simulink model "washout6"  (R2018b)
settings: Solver=VariableStepAuto  StartTime=0.0  StopTime=50  RelTol=1e-3
libraries: simulink x1, fuzblock x1, cstblocks x1
settings Model: Creator=15705  LastModifiedBy=15705

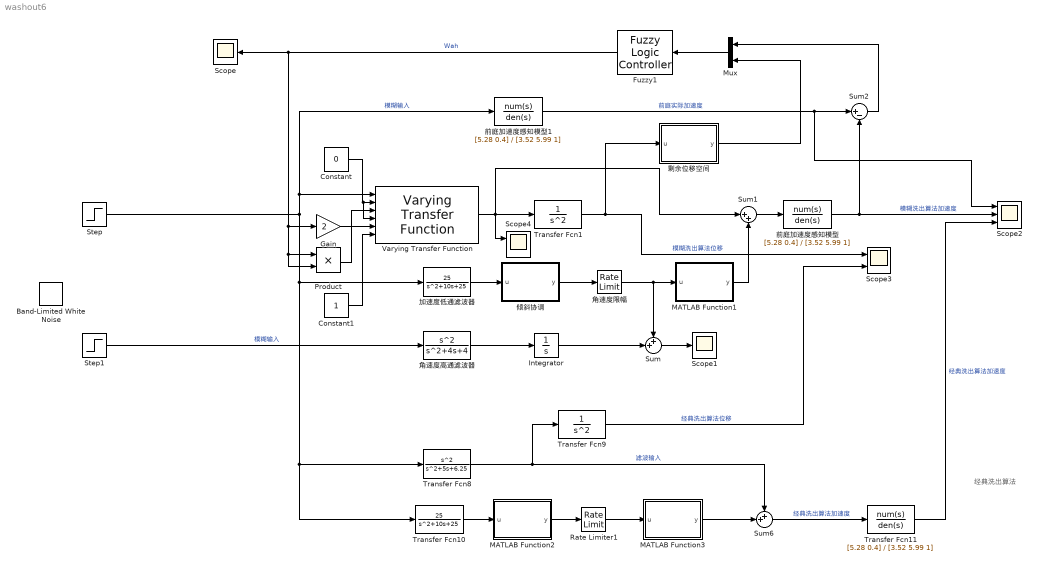
== system washout6 ==
  note: 经典洗出算法
  Band-Limited White Noise : simulink/Sources/Band-Limited White Noise  Cov=[1]  Ts=3  seed=[23341]
  Constant : Constant  Value=0
  Constant1 : Constant
  Fuzzy1 : fuzblock/Fuzzy Logic  Controller  FIS=WahFuzzy  OutputSampleNumber=101  DataType=double  FuzzifiedInputs=off  RuleFiringStrengths=off  RuleOutputs=off  AggregatedOutputs=off  SimulateUsing=Interpreted execution  OutOfRangeInputValueMessage=warning  NoRuleFiredMessage=warning  EmptyOutputFuzzySetMessage=warning
  Gain : Gain  Gain=2
  Integrator : Integrator
  MATLAB Function1 : MATLAB Function  TreatAsAtomicUnit=on
  MATLAB Function2 : MATLAB Function  TreatAsAtomicUnit=on
  MATLAB Function3 : MATLAB Function  TreatAsAtomicUnit=on
  Mux : Mux  Inputs=2
  Product : Product
  Rate Limiter1 : RateLimiter  RisingSlewLimit=0.0628  FallingSlewLimit=-0.0628  SampleTimeMode=inherited
  Scope : Scope
  Scope1 : Scope
  Scope2 : Scope  NumInputPorts=3
  Scope3 : Scope  NumInputPorts=2
  Scope4 : Scope  NumInputPorts=2
  Step : Step  SampleTime=0
  Step1 : Step  SampleTime=0
  Sum : Sum  Inputs=++|
  Sum1 : Sum  Inputs=|++
  Sum2 : Sum  Inputs=|+-
  Sum6 : Sum  Inputs=++|
  Transfer Fcn1 : TransferFcn  Denominator=[1 0 0]
  Transfer Fcn10 : TransferFcn  Numerator=[25]  Denominator=[1 10 25]
  Transfer Fcn11 : TransferFcn  Numerator=[5.28 0.4]  Denominator=[3.52 5.99 1]
  Transfer Fcn8 : TransferFcn  Numerator=[1 0 0]  Denominator=[1 5 6.25]
  Transfer Fcn9 : TransferFcn  Denominator=[1 0 0]
  Varying Transfer Function : cstblocks/Linear Parameter Varying/Varying Transfer Function  N=2
      settings: SourceProductName=Control System Toolbox
  倾斜协调 : MATLAB Function  TreatAsAtomicUnit=on
  前庭加速度感知模型 : TransferFcn  Numerator=[5.28 0.4]  Denominator=[3.52 5.99 1]
  前庭加速度感知模型1 : TransferFcn  Numerator=[5.28 0.4]  Denominator=[3.52 5.99 1]
  剩余位移空间 : MATLAB Function  TreatAsAtomicUnit=on
  加速度低通滤波器 : TransferFcn  Numerator=[25]  Denominator=[1 10 25]
  角速度限幅 : RateLimiter  RisingSlewLimit=0.0628  FallingSlewLimit=-0.0628  SampleTimeMode=inherited
  角速度高通滤波器 : TransferFcn  Numerator=[1 0 0]  Denominator=[1 4 4]
  wires:
  Transfer Fcn10/1 -> MATLAB Function2/1(u)
  MATLAB Function2/1(y) -> Rate Limiter1/1
  Rate Limiter1/1 -> MATLAB Function3/1(u)
  Sum6/1 -> Transfer Fcn11/1  "经典洗出算法加速度"
  Step/1 -> Varying Transfer Function/1, 前庭加速度感知模型1/1, Transfer Fcn10/1, Transfer Fcn8/1, 加速度低通滤波器/1  "模糊输入"
  MATLAB Function3/1(y) -> Sum6/2
  Transfer Fcn8/1 -> Transfer Fcn9/1, Sum6/1  "滤波输入"
  Varying Transfer Function/1 -> Transfer Fcn1/1, Scope4/1, Sum1/1
  Transfer Fcn1/1 -> Scope3/1, 剩余位移空间/1(u)  "模糊洗出算法位移"
  加速度低通滤波器/1 -> 倾斜协调/1(u)
  倾斜协调/1(y) -> 角速度限幅/1
  角速度高通滤波器/1 -> Integrator/1
  Integrator/1 -> Sum/2
  角速度限幅/1 -> MATLAB Function1/1(u), Sum/1
  Sum/1 -> Scope1/1
  Step1/1 -> 角速度高通滤波器/1  "模糊输入"
  MATLAB Function1/1(y) -> Sum1/2
  Sum1/1 -> 前庭加速度感知模型/1
  前庭加速度感知模型/1 -> Sum2/2, Scope2/2  "模糊洗出算法加速度"
  前庭加速度感知模型1/1 -> Scope2/1, Sum2/1  "前庭实际加速度"
  Sum2/1 -> Mux/1
  剩余位移空间/1(y) -> Mux/2
  Mux/1 -> Fuzzy1/1
  Transfer Fcn11/1 -> Scope2/3  "经典洗出算法加速度"
  Transfer Fcn9/1 -> Scope3/2  "经典洗出算法位移"
  Constant/1 -> Varying Transfer Function/4, Varying Transfer Function/2
  Constant1/1 -> Varying Transfer Function/6
  Fuzzy1/1 -> Gain/1, Product/2, Product/1, Scope/1  "Wah"
  Product/1 -> Varying Transfer Function/3
  Gain/1 -> Varying Transfer Function/5

== matlab function washout6/MATLAB Function1 ==
  data: u input; y output
function y = fcn(u)
y=9.8*sin(u);

== matlab function washout6/倾斜协调 ==
  data: u input; y output
function y = fcn(u)
y=asin(u/9.8);

== matlab function washout6/MATLAB Function2 ==
  data: u input; y output
function y = fcn(u)
y=asin(u/9.8);

== matlab function washout6/MATLAB Function3 ==
  data: u input; y output
function y = fcn(u)
y=9.8*sin(u);

== matlab function washout6/剩余位移空间 ==
  data: u input; y output
function y = fcn(u)
if abs(u)<0.2
    y=1-abs(u)/0.2; %剩余空间
else
    y=0
end
